simulink model "Monomagnet_random"  (R2023b)
settings: Solver=FixedStepAuto  StartTime=0.0  StopTime=0.6  FixedStep=0.000001  MaxStep=0.001  RelTol=1e-3
settings Model: Creator=16536  LastModifiedBy=Mitcher
settings SolverCC: ZeroCrossAlgorithm=Adaptive  AlgebraicLoopSolver=TrustRegion  EnableFixedStepZeroCrossing=on
settings DebuggingCC: MaxConsecutiveZCsMsg=warning  IgnoredZcDiagnostic=none
settings ModelReferenceCC: EnableRefExpFcnMdlSchedulingChecks=on
settings SFSimCC: SimTargetLang=C++
settings RTWCC: DLArmComputeVersion=19.05

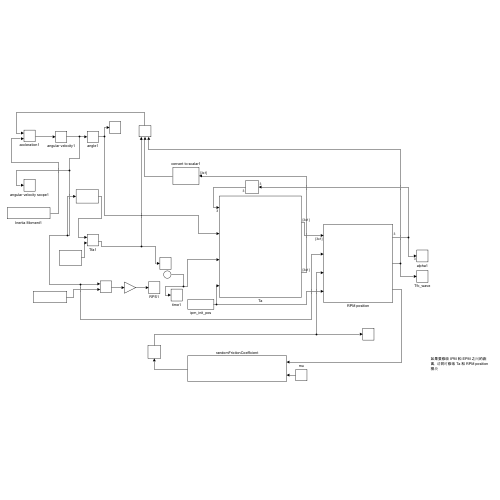
[thumbnail: Simulink's stored preview of the top-level diagram]
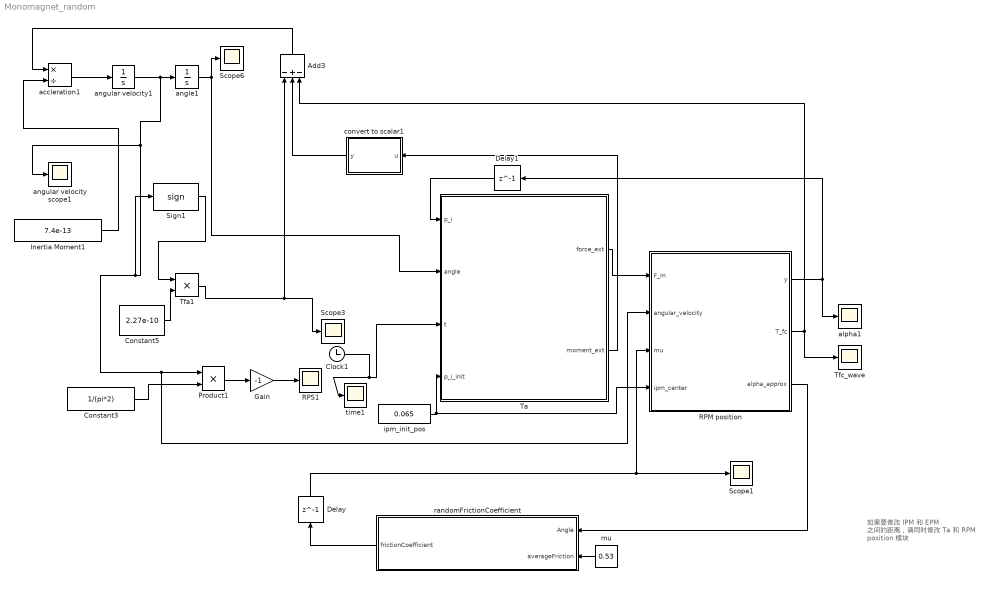
== system Monomagnet_random ==
  note: 如果要修改 IPM 和 EPM 之间的距离，请同时修改 Ta 和 RPM position 模块
  Add3 : Sum  Inputs=-+-
  Clock1 : Clock
  Constant3 : Constant  Value=1/(pi*2)
  Constant5 : Constant  Value=2.27e-10
  Delay : Delay  DelayLength=1
  Delay1 : Delay  DelayLength=1  InitialCondition=[0.05+0.025*cos(0)*10e-3; 0.025*sin(0)*10e-3; 0];  SampleTime=0.001
  Gain : Gain  Gain=-1
  Inertia Moment1 : Constant  Value=7.4e-13
  Product1 : Product
  RPM position : MATLAB Function  TreatAsAtomicUnit=on
  RPS1 : Scope
  Scope1 : Scope
  Scope3 : Scope
  Scope6 : Scope
  Sign1 : Signum
  Ta : MATLAB Function  TreatAsAtomicUnit=on
  Tfa1 : Product  Inputs=**
  Tfc_wave : Scope
  accleration1 : Product  Inputs=*/
  alpha1 : Scope
  angle1 : Integrator
  angular velocity scope1 : Scope
  angular velocity1 : Integrator  InitialCondition=0.0001  LimitOutput=on  UpperSaturationLimit=0.0001  LowerSaturationLimit=-600
  convert to scalar1 : MATLAB Function  TreatAsAtomicUnit=on
  ipm_init_pos : Constant  Value=0.065
  mu : Constant  Value=0.53
  randomFrictionCoefficient : MATLAB Function  TreatAsAtomicUnit=on
  time1 : Scope
  wires:
  Ta/1(force_ext) -> RPM position/1(F_m)
  Delay1/1 -> Ta/1(p_i)
  Ta/2(moment_ext) -> convert to scalar1/1(u)
  RPM position/1(y) -> Delay1/1, alpha1/1
  Add3/1 -> accleration1/1
  Clock1/1 -> Ta/3(t), time1/1
  Constant5/1 -> Tfa1/2
  Sign1/1 -> Tfa1/1
  Product1/1 -> Gain/1
  Constant3/1 -> Product1/2
  accleration1/1 -> angular velocity1/1
  Inertia Moment1/1 -> accleration1/2
  angular velocity1/1 -> angle1/1, Sign1/1, RPM position/2(angular_velocity), Product1/1, angular velocity scope1/1
  angle1/1 -> Ta/2(angle), Scope6/1
  convert to scalar1/1(y) -> Add3/2
  Tfa1/1 -> Scope3/1, Add3/1
  Gain/1 -> RPS1/1
  RPM position/3(alpha_approx) -> randomFrictionCoefficient/1(Angle)
  randomFrictionCoefficient/1(frictionCoefficient) -> Delay/1
  Delay/1 -> Scope1/1, RPM position/3(mu)
  RPM position/2(T_fc) -> Tfc_wave/1, Add3/3
  mu/1 -> randomFrictionCoefficient/2(averageFriction)
  ipm_init_pos/1 -> RPM position/4(ipm_center), Ta/4(p_i_init)

== matlab function Monomagnet_random/RPM position ==
  data: F_m input; y output; T_fc output; angular_velocity input; alpha_approx output; mu input; ipm_center input
function [y, T_fc, alpha_approx] = solve_equation(F_m, angular_velocity, mu, ipm_center)
    m  = 5.9e-6;
    R = 0.525e-3; % 套管半径
    g = 9.8;
    r = 0.5e-3; % 转子半径
    %mu = 0.53; % 摩擦系数
%     mu = 0.5;
    F_mx = F_m(1);
    F_my = F_m(2);
    % 定义方程   
    F_inertial = m * angular_velocity^2 * r;
    equation = @(alpha) (F_my * sin(alpha) + mu * F_my * cos(alpha) - m * g * sin(alpha) - mu * m * g * cos(alpha) - F_inertial * cos(alpha) * sin(alpha) - mu * F_inertial * cos(alpha)^2) - (F_mx * cos(alpha) - mu * F_mx * sin(alpha) - F_inertial * sin(alpha) * cos(alpha) + mu * F_inertial * sin(alpha)^2);  
    % 定义方程的导数
    equationDerivative = @(alpha) (F_my * cos(alpha) - mu * F_my * sin(alpha) - m * g * cos(alpha) + mu * m * g * sin(alpha) + F_inertial * sin(alpha)^2 - mu * F_inertial * sin(alpha) * cos(alpha) + F_inertial * cos(alpha)^2) + (F_mx * sin(alpha) + mu * F_mx * cos(alpha) - F_inertial * cos(alpha) * sin(alpha) - mu * F_inertial * cos(alpha)^2);
    % 初始化初始猜测值
    alpha0 = 0;  % 可根据具体情况选择合适的初始值
    
    % 牛顿法迭代求解方程
    maxIterations = 100;  % 设置最大迭代次数
    tolerance = 0.01745;  % 设置收敛容差,0.01745对应1°
    alpha = alpha0;
    for iteration = 1:maxIterations
        f = equation(alpha);
        df = equationDerivative(alpha);
        delta = f / df;
        alpha = alpha - delta;
        if abs(delta) < tolerance
            break;
        end
    end
    
    F_n = (F_inertial*sin(alpha)-F_mx)/(sin(alpha)+mu * cos(alpha));
%     if F_n > 0
%         T_fc = F_n *r;
%     else
%         T_fc = 0;
%     end
    T_fc = F_n * R;
    alpha_approx = alpha;
    % y = [0.08+(R-r)*cos(alpha); (R-r)*sin(alpha); 0];
    y = [(R-r)*sin(alpha); (ipm_center)-(R-r)*cos(alpha); 0];  % 这个地方修改距离
end

== matlab function Monomagnet_random/randomFrictionCoefficient ==
  settings: updateMethod=DISCRETE
  data: Angle input; frictionCoefficient output; averageFriction input
function frictionCoefficient = calculateFrictionCoefficient(Angle, averageFriction)
    persistent frictionCoefficients;
    persistent theta;
    if isempty(frictionCoefficients)
        % 给定平均摩擦系数
        % averageFriction = 0.53;
        
        % 生成摩擦系数数组，只在第一次调用时生成
        numPoints = 1000; % 假设有1000个接触点
        theta = linspace(0, 2*pi, numPoints); % 生成均匀分布的角度数组
        frictionCoefficients = normrnd(averageFriction, 0.1, numPoints, 1);
        frictionCoefficients = abs(frictionCoefficients);
    end
    if isempty(Angle)
        Angle = 0;
    end
    angle = convertToRadians(Angle);

    % 找到最接近的接触点角度
    [~, index] = min(abs(theta - angle));
    frictionCoefficient = frictionCoefficients(index);
end

function result = convertToRadians(input)
    % 将输入除以 π
    divided = input / pi;
    
    % 将结果限制在 0 到 2π 的范围内
    limited = mod(divided, 2) * pi;
    
    % 如果结果为负数，转换为对应的正数
    result = abs(limited);
end

== matlab function Monomagnet_random/Ta ==
  data: p_i input; force_ext output size=[3,1]; angle input; t input; moment_ext output size=[3;1]; p_i_init input
% 计算磁铁在空间中所受力和力矩 p_i R_i pe re均为 3×1的向量
function [force_ext, moment_ext] = calc_magnet_dipole(p_i, angle, t, p_i_init)

R_i = [cos(angle); sin(angle);0];
    
w_a = 20*pi; %设永磁体转速为10Hz
Re = [cos(w_a*t);sin(w_a*t);0];

%force_ext = zeros(3, 1);
%moment_ext = zeros(3, 1);
pe = [0; 0; 0];
if isempty(p_i)
    % p_i = [0; 55e-3; 0];   % 这个地方修改距离 单位 m
    p_i = [0; p_i_init; 0];
end
mi_norm = 9.15e-4;
me_norm = 9.15e-4*1.25e5;
mu_0 = 4*pi*1e-7; %% 真空磁导率
p = p_i-pe; %% 由磁偶极子指向永磁体的向量[ ]3×1
% p = [-0.0200818832706742;0.0211691934838013;-0.0790695746370514];
p_hat = p/norm(p); 
I = eye(3);

me_vec = 1*(Re/norm(Re))*me_norm;
mi_vec = 1*(R_i/norm(R_i))*mi_norm; %mi_vec是3x1的向量

% mi_vec = [cosd(45);sind(45);0];
h = (1/(4*pi*1^3))*(3*p_hat*(p_hat')-I)*(me_vec);
force_mid =(p'*mi_vec)*me_vec+(p'*me_vec) * mi_vec + (me_vec'*mi_vec-5*(p_hat'*me_vec)*(p_hat'*mi_vec))*p;
force_ext = (3*mu_0/(4*pi*(norm(p))^5))*force_mid;

%mi_vec = mi_vec';h = h';
moment_ext = mu_0*(cross(mi_vec,h));


% energy = -miu0*h'*mi_vec;
end

== matlab function Monomagnet_random/convert to scalar1 ==
  data: u input; y output
function y = fcn(u)

y = u(3);
